simulink model "Motors_PID_Simulink_Main"  (R2019b)
settings: Solver=VariableStepAuto  StartTime=0.0  StopTime=2  FixedStep=0.0001  RelTol=1e-3
values from neighbouring files (symbols this model uses):
  desired_angle_vectors = deg2rad(degree_vectors)    [Motors_Main_Project.m]
  EKb = Kb(3)    [Motors_Main_Project.m]
  EKm = Km(3)    [Motors_Main_Project.m]
  EL = L(3)    [Motors_Main_Project.m]
  SKb = Kb(4)    [Motors_Main_Project.m]
  SKm = Km(4)    [Motors_Main_Project.m]
  SL = L(4)    [Motors_Main_Project.m]
  WKb = Kb(2)    [Motors_Main_Project.m]
  WKm = Km(2)    [Motors_Main_Project.m]
  WL = L(2)    [Motors_Main_Project.m]
undefined symbols (not defined in the file or in its folder): ER, GR, SR
libraries: cstblocks x4
settings Model: Creator=harsh  LastModifiedBy=debby

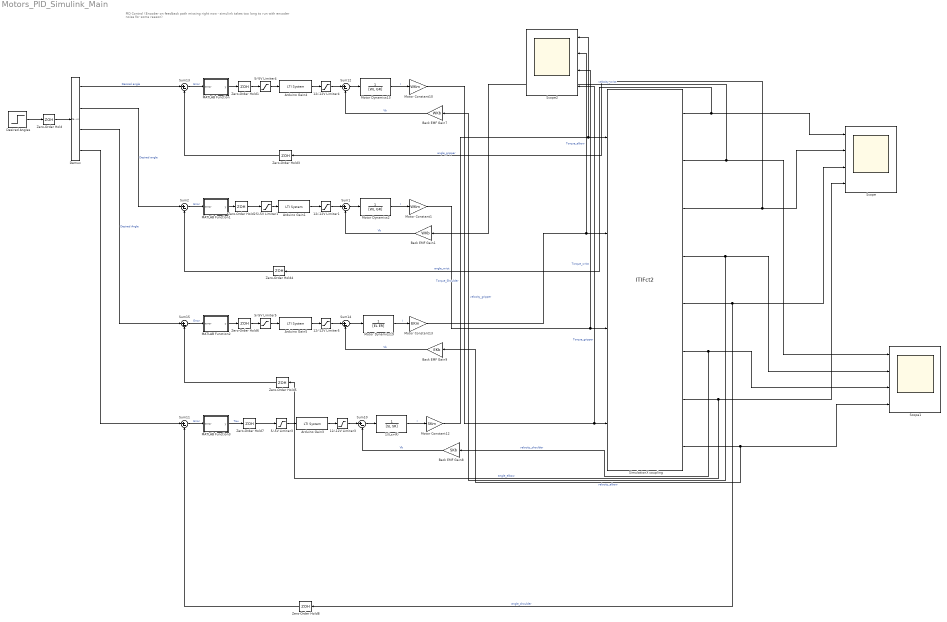
== system Motors_PID_Simulink_Main ==
  note: PID Control
      | (Encoder on feedback path missing right now - simulink takes too long to run with encoder noise for some reason)
  1/(Ls+R) : TransferFcn  Denominator=[SL SR]
  12/-12V Limiter{1,3..5} (4 alike) : Saturate  UpperLimit=12  LowerLimit=-12
  5/-5V Limiter{1,3..5} (4 alike) : Saturate  UpperLimit=5  LowerLimit=-5
  Arduino Gain1 : cstblocks/LTI System  sys=WOPAMP  IC=[]
  Arduino Gain3 : cstblocks/LTI System  sys=SOPAMP  IC=[]
  Arduino Gain4 : cstblocks/LTI System  sys=GOPAMP  IC=[]
  Arduino Gain5 : cstblocks/LTI System  sys=EOPAMP  IC=[]
  Back EMF Gain1 : Gain  Gain=WKb
  Back EMF Gain7 : Gain  Gain=WKb
  Back EMF Gain8 : Gain  Gain=SKb
  Back EMF Gain9 : Gain  Gain=EKb
  Demux : Demux
  "Desired Angles " : Step  Time=0.1  After=desired_angle_vectors  SampleTime=0
  MATLAB Function : MATLAB Function  TreatAsAtomicUnit=on
  MATLAB Function1 : MATLAB Function  TreatAsAtomicUnit=on
  MATLAB Function2 : MATLAB Function  TreatAsAtomicUnit=on
  MATLAB Function3 : MATLAB Function  TreatAsAtomicUnit=on
  Motor Constant1 : Gain  Gain=WKm
  Motor Constant10 : Gain  Gain=WKm
  Motor Constant12 : Gain  Gain=SKm
  Motor Constant13 : Gain  Gain=EKm
  Motor Dynamics13 : TransferFcn  Denominator=[WL GR]
  Motor Dynamics19 : TransferFcn  Denominator=[EL ER]
  Motor Dynamics2 : TransferFcn  Denominator=[WL GR]
  Scope : Scope  NumInputPorts=4
  Scope1 : Scope  NumInputPorts=4
  Scope2 : Scope  NumInputPorts=4
  SimulationX coupling : S-Function  FunctionName=ITIFct2  Parameters=ip, port, ts, nIn, nOut  SFunctionDeploymentMode=off  EnableBusSupport=off  mask{ip='localhost', port=1025, ts=0.001, nIn=4, nOut=8}
      mask prompts: ip "Address: ip"; port "Port Number: port [-]"; ts "Communication Step Size: ts [s]"; nIn "Input Vector Dimension (to SimulationX): nIn [-]"; nOut "Output Vector Dimension (from SimulationX): nOut [-]"
      mask help: Coupling Element
  Sum{1..2,10..15} (8 alike) : Sum  Inputs=|+-
  Zero-Order Hold{,1,3..8} (8 alike) : ZeroOrderHold  SampleTime=0.0001
  Zero-Order Hold2 : ZeroOrderHold  SampleTime=-1
  wires:
  "Desired Angles "/1 -> Zero-Order Hold/1
  5/-5V Limiter4/1 -> Arduino Gain4/1
  Arduino Gain4/1 -> 12/-12V Limiter4/1
  Back EMF Gain7/1 -> Sum12/2  "Vb"
  Sum12/1 -> Motor Dynamics13/1
  Demux/1 -> Sum13/1  "Desired angle"
  12/-12V Limiter4/1 -> Sum12/1
  Motor Dynamics13/1 -> Motor Constant10/1  "I"
  Motor Constant10/1 -> Scope2/4, SimulationX coupling/4  "Torque_gripper"
  Sum13/1 -> MATLAB Function/1(error)  "Error"
  Sum2/1 -> MATLAB Function1/1(error)  "Error"
  12/-12V Limiter1/1 -> Sum1/1
  Motor Dynamics2/1 -> Motor Constant1/1  "I"
  Sum1/1 -> Motor Dynamics2/1
  5/-5V Limiter1/1 -> Arduino Gain1/1
  Back EMF Gain1/1 -> Sum1/2  "Vb"
  Arduino Gain1/1 -> 12/-12V Limiter1/1
  Demux/2 -> Sum2/1  "Desired angle"
  MATLAB Function2/1(y) -> Zero-Order Hold6/1
  Sum15/1 -> MATLAB Function2/1(error)  "Error"
  Motor Dynamics19/1 -> Motor Constant13/1  "I"
  Motor Constant13/1 -> Scope2/2, SimulationX coupling/2  "Torque_elbow"
  12/-12V Limiter5/1 -> Sum14/1
  Sum14/1 -> Motor Dynamics19/1
  5/-5V Limiter5/1 -> Arduino Gain5/1
  Back EMF Gain9/1 -> Sum14/2  "Vb"
  Arduino Gain5/1 -> 12/-12V Limiter5/1
  Demux/3 -> Sum15/1  "Desired Angle"
  Back EMF Gain8/1 -> Sum10/2  "Vb"
  Motor Constant12/1 -> SimulationX coupling/1, Scope2/1  "Torque_Shoulder"
  5/-5V Limiter3/1 -> Arduino Gain3/1
  Arduino Gain3/1 -> 12/-12V Limiter3/1
  1/(Ls+R)/1 -> Motor Constant12/1  "I"
  12/-12V Limiter3/1 -> Sum10/1
  MATLAB Function3/1(y) -> Zero-Order Hold7/1  "Tau"
  Sum11/1 -> MATLAB Function3/1(error)  "Error"
  Sum10/1 -> 1/(Ls+R)/1
  Demux/4 -> Sum11/1
  MATLAB Function1/1(y) -> Zero-Order Hold2/1
  MATLAB Function/1(y) -> Zero-Order Hold1/1
  Zero-Order Hold/1 -> Demux/1
  Zero-Order Hold1/1 -> 5/-5V Limiter4/1
  Zero-Order Hold2/1 -> 5/-5V Limiter1/1
  Zero-Order Hold3/1 -> Sum13/2
  Zero-Order Hold4/1 -> Sum2/2
  Zero-Order Hold5/1 -> Sum15/2
  Zero-Order Hold6/1 -> 5/-5V Limiter5/1
  Zero-Order Hold7/1 -> 5/-5V Limiter3/1
  Zero-Order Hold8/1 -> Sum11/2
  SimulationX coupling/2 -> Back EMF Gain1/1, Scope1/1  "velocity_wrist"
  SimulationX coupling/1 -> Zero-Order Hold4/1, Scope/1  "angle_wrist"
  SimulationX coupling/3 -> Zero-Order Hold3/1, Scope/2  "angle_gripper"
  SimulationX coupling/4 -> Back EMF Gain7/1, Scope1/2  "velocity_gripper"
  Motor Constant1/1 -> Scope2/3, SimulationX coupling/3  "Torque_wrist"
  SimulationX coupling/5 -> Zero-Order Hold8/1, Scope/3  "angle_shoulder"
  SimulationX coupling/6 -> Back EMF Gain8/1, Scope1/3  "velocity_shoulder"
  SimulationX coupling/7 -> Zero-Order Hold5/1, Scope/4  "angle_elbow"
  SimulationX coupling/8 -> Back EMF Gain9/1, Scope1/4  "velocity_elbow"

== matlab function Motors_PID_Simulink_Main/MATLAB Function1 ==
  settings: updateMethod=DISCRETE
  data: error input; y output
function y = fcn(error)

persistent previous_error;                  %previous error = current error for next iteration, initially set to 0;
persistent Ki_output;                        %need as persistent variable for Ki_output = Ki_output + (...)
persistent ept;                             %constant vector of exponentials (p*e^(-p*n*Ts)) where n = 1.....#of samples we want to average
persistent unweighted_differential_outputs;  %vector used for dot product with ept, shifted at each cycle. 

if isempty(previous_error)
    previous_error = 0;
end

%Trial values for testing against Built in PID block
Kp = 7.3697;
Ki = 24.525;
Kd = 0.04744;

Ts = 0.0001;    %Controller frequency from Arduino assumed to be 10kHz.

%--------P controller part------------------
Kp_output = Kp*error;    

%---------I controller part-----------------

%Initializing Ki_output
if isempty(Ki_output)
    Ki_output = 0;
end

Ki_output = Ki_output + Ki*[(error + previous_error)/2]*Ts; %cumulative areas of trapeziums

%----------D controller part----------------
controlfreq = 10000; %Hz
filter_pole = 5000;  %big pole because we don't care much about averaging but we do care a lot about delay. (signal is not noisy)
n = 4*controlfreq/filter_pole;  %We are averaging 80 samples in this example


%Now, we initialize the ept vector (will remain constant valued throughout the program)
if isempty(ept)
    ept = zeros(1,n);
    for i = 1:n
        ept(i) = filter_pole*1.132*exp(-filter_pole*i*Ts);
    end
    %We want Ts*sum(ept) = 1 but this is not the case normally, so we have to scale the ept such that we get a sum
    %of 1. To account for discretization error, we scale it by multiplying it by 1.132 in this example. 
end

if isempty(unweighted_differential_outputs)
    unweighted_differential_outputs = zeros(1,n);
end 

unweighted_differential_outputs(1) = (error - previous_error); 
filtered_derivative = dot(ept,unweighted_differential_outputs);

Kd_output = Kd*filtered_derivative;

n2 = n+1; %n2 = 9
for count = 1:(n-1) %1:7 in this example
    unweighted_differential_outputs(n2-count) = unweighted_differential_outputs(n2 - count - 1);    %shift values by one index, and in next loop calculate one more new slope at index 1 (starting index)
end 

y = Kp_output + Ki_output + Kd_output;

previous_error = error; %this will help us move on to get new values for Ki and Kd

end

== matlab function Motors_PID_Simulink_Main/MATLAB Function ==
  settings: updateMethod=DISCRETE
  data: error input; y output
function y = fcn(error)

persistent previous_error;                  %previous error = current error for next iteration, initially set to 0;
persistent Ki_output;                        %need as persistent variable for Ki_output = Ki_output + (...)
persistent ept;                             %constant vector of exponentials (p*e^(-p*n*Ts)) where n = 1.....#of samples we want to average
persistent unweighted_differential_outputs;  %vector used for dot product with ept, shifted at each cycle. 

if isempty(previous_error)
    previous_error = 0;
end

%Trial values for testing against Built in PID block
Kp = 7.3697;
Ki = 24.525;
Kd = 0.04744;

Ts = 0.0001;    %Controller frequency from Arduino assumed to be 10kHz.

%--------P controller part------------------
Kp_output = Kp*error;    

%---------I controller part-----------------

%Initializing Ki_output
if isempty(Ki_output)
    Ki_output = 0;
end

Ki_output = Ki_output + Ki*[(error + previous_error)/2]*Ts; %cumulative areas of trapeziums

%----------D controller part----------------
controlfreq = 10000; %Hz
filter_pole = 5000;  %big pole because we don't care much about averaging but we do care a lot about delay. (signal is not noisy)
n = 4*controlfreq/filter_pole;  %We are averaging 80 samples in this example


%Now, we initialize the ept vector (will remain constant valued throughout the program)
if isempty(ept)
    ept = zeros(1,n);
    for i = 1:n
        ept(i) = filter_pole*1.132*exp(-filter_pole*i*Ts);
    end
    %We want Ts*sum(ept) = 1 but this is not the case normally, so we have to scale the ept such that we get a sum
    %of 1. To account for discretization error, we scale it by multiplying it by 1.132 in this example. 
end

if isempty(unweighted_differential_outputs)
    unweighted_differential_outputs = zeros(1,n);
end 

unweighted_differential_outputs(1) = (error - previous_error); 
filtered_derivative = dot(ept,unweighted_differential_outputs);

Kd_output = Kd*filtered_derivative;

n2 = n+1; %n2 = 9
for count = 1:(n-1) %1:7 in this example
    unweighted_differential_outputs(n2-count) = unweighted_differential_outputs(n2 - count - 1);    %shift values by one index, and in next loop calculate one more new slope at index 1 (starting index)
end 

y = Kp_output + Ki_output + Kd_output;

previous_error = error; %this will help us move on to get new values for Ki and Kd

end

== matlab function Motors_PID_Simulink_Main/MATLAB Function2 ==
  settings: updateMethod=DISCRETE
  data: error input; y output
function y = fcn(error)

persistent previous_error;                  %previous error = current error for next iteration, initially set to 0;
persistent Ki_output;                        %need as persistent variable for Ki_output = Ki_output + (...)
persistent ept;                             %constant vector of exponentials (p*e^(-p*n*Ts)) where n = 1.....#of samples we want to average
persistent unweighted_differential_outputs;  %vector used for dot product with ept, shifted at each cycle. 

if isempty(previous_error)
    previous_error = 0;
end

%Trial values for testing against Built in PID block
Kp = 7.3697;
Ki = 24.525;
Kd = 0.04744;

Ts = 0.0001;    %Controller frequency from Arduino assumed to be 10kHz.

%--------P controller part------------------
Kp_output = Kp*error;    

%---------I controller part-----------------

%Initializing Ki_output
if isempty(Ki_output)
    Ki_output = 0;
end

Ki_output = Ki_output + Ki*[(error + previous_error)/2]*Ts; %cumulative areas of trapeziums

%----------D controller part----------------
controlfreq = 10000; %Hz
filter_pole = 5000;  %big pole because we don't care much about averaging but we do care a lot about delay. (signal is not noisy)
n = 4*controlfreq/filter_pole;  %We are averaging 80 samples in this example


%Now, we initialize the ept vector (will remain constant valued throughout the program)
if isempty(ept)
    ept = zeros(1,n);
    for i = 1:n
        ept(i) = filter_pole*1.132*exp(-filter_pole*i*Ts);
    end
    %We want Ts*sum(ept) = 1 but this is not the case normally, so we have to scale the ept such that we get a sum
    %of 1. To account for discretization error, we scale it by multiplying it by 1.132 in this example. 
end

if isempty(unweighted_differential_outputs)
    unweighted_differential_outputs = zeros(1,n);
end 

unweighted_differential_outputs(1) = (error - previous_error); 
filtered_derivative = dot(ept,unweighted_differential_outputs);

Kd_output = Kd*filtered_derivative;

n2 = n+1; %n2 = 9
for count = 1:(n-1) %1:7 in this example
    unweighted_differential_outputs(n2-count) = unweighted_differential_outputs(n2 - count - 1);    %shift values by one index, and in next loop calculate one more new slope at index 1 (starting index)
end 

y = Kp_output + Ki_output + Kd_output;

previous_error = error; %this will help us move on to get new values for Ki and Kd

end

== matlab function Motors_PID_Simulink_Main/MATLAB Function3 ==
  settings: updateMethod=DISCRETE
  data: error input; y output
function y = fcn(error)

persistent previous_error;                  %previous error = current error for next iteration, initially set to 0;
persistent Ki_output;                        %need as persistent variable for Ki_output = Ki_output + (...)
persistent ept;                             %constant vector of exponentials (p*e^(-p*n*Ts)) where n = 1.....#of samples we want to average
persistent unweighted_differential_outputs;  %vector used for dot product with ept, shifted at each cycle. 

if isempty(previous_error)
    previous_error = 0;
end

%Trial values for testing against Built in PID block
Kp = 7.3697;
Ki = 24.525;
Kd = 0.04744;

Ts = 0.0001;    %Controller frequency from Arduino assumed to be 10kHz.

%--------P controller part------------------
Kp_output = Kp*error;    

%---------I controller part-----------------

%Initializing Ki_output
if isempty(Ki_output)
    Ki_output = 0;
end

Ki_output = Ki_output + Ki*[(error + previous_error)/2]*Ts; %cumulative areas of trapeziums

%----------D controller part----------------
controlfreq = 10000; %Hz
filter_pole = 5000;  %big pole because we don't care much about averaging but we do care a lot about delay. (signal is not noisy)
n = 4*controlfreq/filter_pole;  %We are averaging 80 samples in this example


%Now, we initialize the ept vector (will remain constant valued throughout the program)
if isempty(ept)
    ept = zeros(1,n);
    for i = 1:n
        ept(i) = filter_pole*1.132*exp(-filter_pole*i*Ts);
    end
    %We want Ts*sum(ept) = 1 but this is not the case normally, so we have to scale the ept such that we get a sum
    %of 1. To account for discretization error, we scale it by multiplying it by 1.132 in this example. 
end

if isempty(unweighted_differential_outputs)
    unweighted_differential_outputs = zeros(1,n);
end 

unweighted_differential_outputs(1) = (error - previous_error); 
filtered_derivative = dot(ept,unweighted_differential_outputs);

Kd_output = Kd*filtered_derivative;

n2 = n+1; %n2 = 9
for count = 1:(n-1) %1:7 in this example
    unweighted_differential_outputs(n2-count) = unweighted_differential_outputs(n2 - count - 1);    %shift values by one index, and in next loop calculate one more new slope at index 1 (starting index)
end 

y = Kp_output + Ki_output + Kd_output;

previous_error = error; %this will help us move on to get new values for Ki and Kd

end
